simulink model "chap3_8sim"  (Simulink 8.3)
settings: Solver=ode45  StartTime=0.0  StopTime=10  RelTol=1e-3
settings Model: Creator=ljk  LastModifiedBy=Administrator  ExtModeTrigMode=oneshot  ExtModeArmWhenConnect=off
settings DataIOCC: LimitDataPoints=off  SignalLoggingName=sigsOut
settings OptimizationCC: BooleanDataType=off  ExpressionDepthLimit=2147483647
settings DebuggingCC: SaveWithParameterizedLinksMsg=none  SignalResolutionControl=TryResolveAllWithWarning  SolverPrmCheckMsg=none  MultiTaskDSMMsg=warning  MultiTaskCondExecSysMsg=none  FcnCallInpInsideContextMsg=UseLocalSettings
settings HardwareCC: TargetUnknown=on
settings RTWCC: IncludeERTFirstTime=on

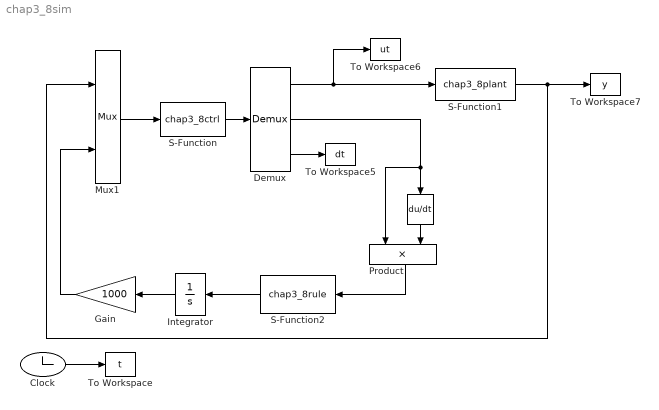
== system chap3_8sim ==
  "  " : Derivative
  Clock : Clock
  Demux : Demux  Outputs=3
  Gain : Gain  Gain=1000  SaturateOnIntegerOverflow=on  OutDataTypeStr=Inherit: Same as input  ParamDataTypeStr=Inherit: Same as input
  Integrator : Integrator
  Mux1 : Mux  Inputs=2
  Product : Product  SaturateOnIntegerOverflow=on  InputSameDT=on  OutDataTypeStr=Inherit: Same as first input
  S-Function : S-Function  FunctionName=chap3_8ctrl  EnableBusSupport=off
  S-Function1 : S-Function  FunctionName=chap3_8plant  EnableBusSupport=off
  S-Function2 : S-Function  FunctionName=chap3_8rule  EnableBusSupport=off
  To Workspace : ToWorkspace  VariableName=t  SampleTime=-1
  To Workspace5 : ToWorkspace  VariableName=dt  SampleTime=-1
  To Workspace6 : ToWorkspace  VariableName=ut  SampleTime=-1
  To Workspace7 : ToWorkspace  VariableName=y  SampleTime=-1
  wires:
  Mux1/1 -> S-Function/1
  S-Function/1 -> Demux/1
  Demux/2 -> "  "/1, Product/1
  Demux/1 -> S-Function1/1, To Workspace6/1
  S-Function2/1 -> Integrator/1
  Gain/1 -> Mux1/2
  Integrator/1 -> Gain/1
  Demux/3 -> To Workspace5/1
  S-Function1/1 -> To Workspace7/1, Mux1/1
  Product/1 -> S-Function2/1
  Clock/1 -> To Workspace/1
  "  "/1 -> Product/2
